simulink model "PlantaTFG"  (R2021b)
settings: Solver=FixedStepAuto  StartTime=0.0  StopTime=30  FixedStep=0.001  RelTol=1e-3
values from neighbouring files (symbols this model uses):
  K = 50    [TFG_Preload.m]
  Kpot = 1.688    [TFG_Preload.m]
  Ktac = 0.01338    [TFG_Preload.m]
  tau = 0.255    [TFG_Preload.m]
undefined symbols (not defined in the file or in its folder): Kd, Ki, Kp
libraries: simulink x1
settings Model: Creator=FactCore  LastModifiedBy=FactCore

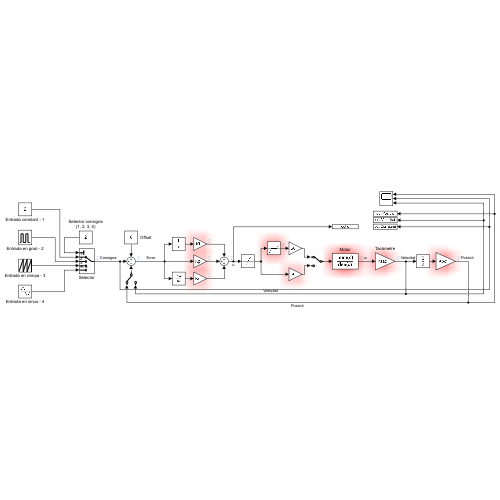
[thumbnail: Simulink's stored preview of the top-level diagram]
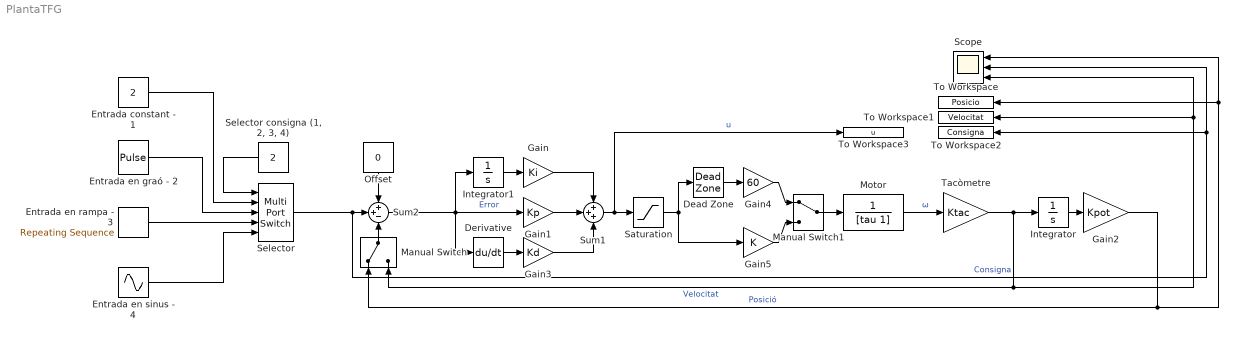
== system PlantaTFG ==
  Dead Zone : DeadZone  LowerValue=Vdi  UpperValue=Vds  SaturateOnIntegerOverflow=on
  Derivative : Derivative
  Entrada constant - 1 : Constant  Value=2
  Entrada en graó - 2 : DiscretePulseGenerator  PulseType=Time based  Amplitude=3  Period=10  PulseWidth=50
  Entrada en rampa - 3 : simulink/Sources/Repeating Sequence  rep_seq_t=[0 10]  rep_seq_y=[0 0.5]
  Entrada en sinus - 4 : Sin  Amplitude=5  Frequency=2*pi*0.5  SampleTime=0
  Gain : Gain  Gain=Ki
  Gain1 : Gain  Gain=Kp
  Gain2 : Gain  Gain=Kpot
  Gain3 : Gain  Gain=Kd
  Gain4 : Gain  Gain=60
  Gain5 : Gain  Gain=K
  Integrator : Integrator
  Integrator1 : Integrator
  Manual Switch : ManualSwitch
  Manual Switch1 : ManualSwitch
  Motor : TransferFcn  Denominator=[tau 1]
  Offset : Constant  Value=0
  Saturation : Saturate  UpperLimit=5  LowerLimit=-5
  Scope : Scope  NumInputPorts=3
  Selector : MultiPortSwitch  Inputs=4  OutDataTypeStr=single
  "Selector consigna (1, 2, 3, 4)" : Constant  Value=2
  Sum1 : Sum  Inputs=+++
  Sum2 : Sum  Inputs=++-
  Tacòmetre : Gain  Gain=Ktac
  To Workspace : ToWorkspace  VariableName=Posicio  SaveFormat=Timeseries  SampleTime=-1
  To Workspace1 : ToWorkspace  VariableName=Velocitat  SaveFormat=Timeseries  SampleTime=-1
  To Workspace2 : ToWorkspace  VariableName=Consigna  SaveFormat=Timeseries  SampleTime=-1
  To Workspace3 : ToWorkspace  VariableName=u  SaveFormat=Timeseries  SampleTime=-1
  wires:
  Motor/1 -> Tacòmetre/1  "ω"
  Sum2/1 -> Derivative/1, Integrator1/1, Gain1/1  "Error"
  Tacòmetre/1 -> To Workspace1/1, Scope/3, Manual Switch/2, Integrator/1  "Velocitat"
  Integrator/1 -> Gain2/1
  Integrator1/1 -> Gain/1
  Derivative/1 -> Gain3/1
  Gain/1 -> Sum1/1
  Gain3/1 -> Sum1/3
  Gain1/1 -> Sum1/2
  Sum1/1 -> To Workspace3/1, Saturation/1  "u"
  "Selector consigna (1, 2, 3, 4)"/1 -> Selector/1
  Entrada en graó - 2/1 -> Selector/3
  Entrada en rampa - 3/1 -> Selector/4
  Entrada constant - 1/1 -> Selector/2
  Selector/1 -> Scope/2, To Workspace2/1, Sum2/2  "Consigna"
  Entrada en sinus - 4/1 -> Selector/5
  Offset/1 -> Sum2/1
  Manual Switch/1 -> Sum2/3
  Gain2/1 -> Manual Switch/1, To Workspace/1, Scope/1  "Posició"
  Manual Switch1/1 -> Motor/1
  Saturation/1 -> Dead Zone/1, Gain5/1
  Gain5/1 -> Manual Switch1/2
  Dead Zone/1 -> Gain4/1
  Gain4/1 -> Manual Switch1/1
